simulink model "sampleModel356"  (R2021b)
settings: Solver=VariableStepAuto  StartTime=0.0  StopTime=10.0  RelTol=1e-3
libraries: simulink x5, slpidlib x1
settings Model: Creator=user  LastModifiedBy=user

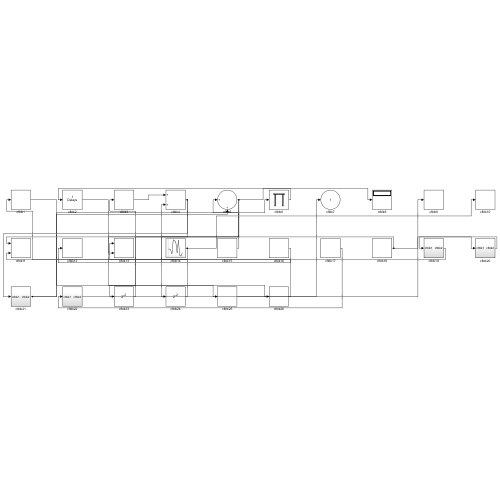
[thumbnail: Simulink's stored preview of the top-level diagram]
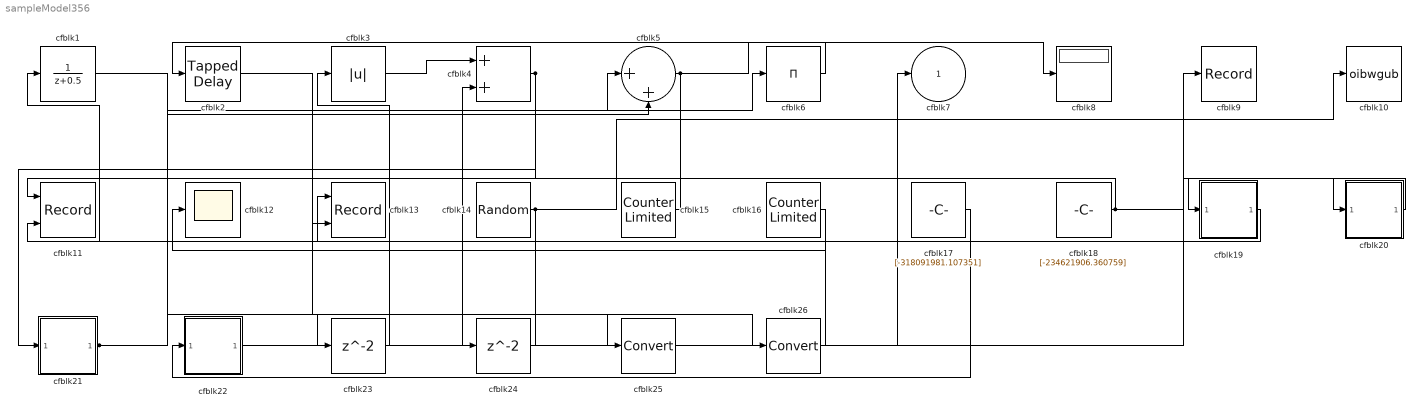
== system sampleModel356 ==
  cfblk1 : DiscreteTransferFcn  SampleTime=1
  cfblk10 : ToWorkspace  VariableName=oibwgub  SaveFormat=Timeseries  SampleTime=-1
  cfblk11 : Record  FileSettingsInternal="{\"entries\":[{\"content\":{\"excelSettings\":{\"content\":{},\"type\":\"Streamout.ExcelSettings\"}},\"type\":\"Streamout.FileSettingStorage\",\"uuid\":\"f7cf1135-fab7-49b0-b509-b4096393f572\"}],\"packageUris\":[\"http://schema.mathworks.com/mf0/streamout_blocks/R2020a\"],\"version\":\"1.0\"}"  Layout=[1 1]  SignalsInternal="{\"entries\":[{\"content\":{\"signals\":[{\"content\":{\"blockPath\":[\"sampleModel356/cfblk11\"],\"channel\":[],\"dimensions\":[1],\"domain\":\"sampleModel356/cfblk11\",\"lineColor\":\"#a2142f\",\"plots\":[1],\"port\":1,\"sid\":[\"\"],\"signalID\":14870,\"signalName\":\"cfblk18\"},\"type\":\"RecordBlkView.Signal\",\"uuid\":\"d168b0b0-4f10-46dc-9af9-509f06b761f4\"},{\"content\":{\"blockPath\":[\"sampleModel356/cfblk11\"],\"channel\":[],\"dimensions\":[1],\"domain\":\"sampleModel356/cfblk11\",\"lineColor\":\"#139fff\",\"plots\":[1],\"port\":2,\"sid\":[\"\"],\"signalID\":14874,\"signalName\":\"cfblk19\"},\"type\":\"RecordBlkView.Signal\",\"uuid\":\"3ec3915b-5336-4778-a6a6-2cfbcdc7d7d8\"}]},\"type\":\"RecordBlkView.InputSignals\",\"uuid\":\"4694ec6d-5d00-4abc-8da0-1736562e4cc9\"}],\"packageUris\":[\"http://schema.mathworks.com/mf0/streamout_blocks/R2020a\"],\"version\":\"1.0\"}"  VisualizationBindings="{\"xyplotplugin\":{\"info\":[{\"series\":[{\"bindingParametersList\":[{\"parameter\":\"X-Axis\",\"signalID\":14870,\"signalName\":\"cfblk18\"},{\"parameter\":\"Y-Axis\",\"signalID\":14874,\"signalName\":\"cfblk19\"}],\"seriesID\":13210}],\"subplotID\":1}]}}"  CompatibilityTag=XY
  cfblk12 : Scope
  cfblk13 : Record  FileSettingsInternal="{\"entries\":[{\"content\":{\"excelSettings\":{\"content\":{},\"type\":\"Streamout.ExcelSettings\"}},\"type\":\"Streamout.FileSettingStorage\",\"uuid\":\"1e1e8cce-afe3-4879-8cf3-0e8c36288c66\"}],\"packageUris\":[\"http://schema.mathworks.com/mf0/streamout_blocks/R2020a\"],\"version\":\"1.0\"}"  Layout=[1 1]  SignalsInternal="{\"entries\":[{\"content\":{\"signals\":[{\"content\":{\"blockPath\":[\"sampleModel356/cfblk13\"],\"channel\":[],\"dimensions\":[1],\"domain\":\"sampleModel356/cfblk13\",\"lineColor\":\"#a2142f\",\"plots\":[1],\"port\":1,\"sid\":[\"\"],\"signalID\":14858,\"signalName\":\"cfblk14\"},\"type\":\"RecordBlkView.Signal\",\"uuid\":\"6a327e09-5034-4fe2-a7e3-7112f60d3f56\"},{\"content\":{\"blockPath\":[\"sampleModel356/cfblk13\"],\"channel\":[],\"dimensions\":[1],\"domain\":\"sampleModel356/cfblk13\",\"lineColor\":\"#139fff\",\"plots\":[1],\"port\":2,\"sid\":[\"\"],\"signalID\":14862,\"signalName\":\"cfblk4\"},\"type\":\"RecordBlkView.Signal\",\"uuid\":\"5deca270-7dad-429e-a242-3b5b02cfe700\"}]},\"type\":\"RecordBlkView.InputSignals\",\"uuid\":\"a51ef856-a68c-416b-b2a1-fe280d763758\"}],\"packageUris\":[\"http://schema.mathworks.com/mf0/streamout_blocks/R2020a\"],\"version\":\"1.0\"}"  VisualizationBindings="{\"xyplotplugin\":{\"info\":[{\"series\":[{\"bindingParametersList\":[{\"parameter\":\"X-Axis\",\"signalID\":14858,\"signalName\":\"cfblk14\"},{\"parameter\":\"Y-Axis\",\"signalID\":14862,\"signalName\":\"cfblk4\"}],\"seriesID\":15766}],\"subplotID\":1}]}}"  CompatibilityTag=XY
  cfblk14 : RandomNumber  Mean=[15872.946615]  Variance=[24959.344930]  Seed=[933413514.000000]  SampleTime=0.1
  cfblk15 : simulink/Sources/Counter Limited  uplimit=[477.000000]  tsamp=-1
  cfblk16 : simulink/Sources/Counter Limited  uplimit=[515.000000]  tsamp=-1
  cfblk17 : Constant  Value=[-318091981.107351]  SampleTime=1
  cfblk18 : Constant  Value=[-234621906.360759]  SampleTime=1
  cfblk19 : Subsystem
  cfblk2 : simulink/Discrete/Tapped Delay  vinit=0.0  samptime=-1  NumDelays=1  DelayOrder=Oldest  includeCurrent=off
  cfblk20 : Subsystem
  cfblk21 : Subsystem
  cfblk22 : Subsystem
  cfblk23 : Delay  SampleTime=1
  cfblk24 : Delay  SampleTime=1
  cfblk25 : DataTypeConversion
  cfblk26 : DataTypeConversion
  cfblk3 : Abs
  cfblk4 : Sum
  cfblk5 : Sum  Inputs=|++
  cfblk6 : Product  Inputs=*
  cfblk8 : Display
  cfblk9 : Record  FileSettingsInternal="{\"entries\":[{\"content\":{\"excelSettings\":{\"content\":{},\"type\":\"Streamout.ExcelSettings\"}},\"type\":\"Streamout.FileSettingStorage\",\"uuid\":\"394831a3-6f16-480d-90e3-9806f58ee700\"}],\"packageUris\":[\"http://schema.mathworks.com/mf0/streamout_blocks/R2020a\"],\"version\":\"1.0\"}"  SignalsInternal="{\"entries\":[{\"content\":{\"signals\":[{\"content\":{\"blockPath\":[\"sampleModel356/cfblk9\"],\"channel\":[],\"dimensions\":[1],\"domain\":\"sampleModel356/cfblk9\",\"lineColor\":\"#edb120\",\"plots\":[1],\"port\":1,\"sid\":[\"\"],\"signalID\":14866,\"signalName\":\"cfblk25\"},\"type\":\"RecordBlkView.Signal\",\"uuid\":\"7e7b1933-ec16-40c2-a7dc-3907081fd54a\"}]},\"type\":\"RecordBlkView.InputSignals\",\"uuid\":\"25d2bbb5-58e4-4035-93b0-d4b8c4893eb6\"}],\"packageUris\":[\"http://schema.mathworks.com/mf0/streamout_blocks/R2020a\"],\"version\":\"1.0\"}"  VisualizationBindings="{\"sparklinesplugin\":{\"info\":[{\"bindingParametersList\":[],\"subplotID\":1}]}}"
  cfblk7 : Outport
  wires:
  cfblk18/1 -> cfblk11/1, cfblk20/1(cfblk1)
  cfblk6/1 -> cfblk2/1
  cfblk3/1 -> cfblk4/1
  cfblk22/1(cfblk2) -> cfblk7/1
  cfblk14/1 -> cfblk13/1, cfblk10/1
  cfblk17/1 -> cfblk22/1(cfblk1)
  cfblk4/1 -> cfblk21/1(cfblk1), cfblk13/2
  cfblk5/1 -> cfblk8/1, cfblk23/1, cfblk24/1
  cfblk20/1(cfblk2) -> cfblk19/1(cfblk1)
  cfblk16/1 -> cfblk12/1
  cfblk21/1(cfblk2) -> cfblk6/1, cfblk5/2
  cfblk15/1 -> cfblk5/1
  cfblk19/1(cfblk2) -> cfblk11/2
  cfblk23/1 -> cfblk3/1
  cfblk24/1 -> cfblk4/2
  cfblk1/1 -> cfblk25/1
  cfblk25/1 -> cfblk9/1
  cfblk2/1 -> cfblk26/1
  cfblk26/1 -> cfblk1/1

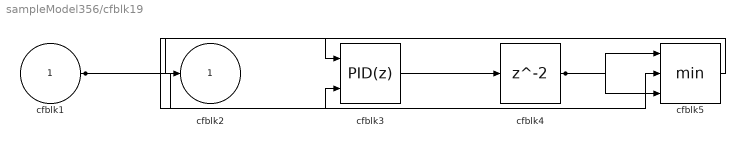
== system sampleModel356/cfblk19 ==
  cfblk1 : Inport
  cfblk3 : slpidlib/PID Controller (2DOF)  Controller=PID  Form=Parallel  TimeDomain=Discrete-time  UseExternalTs=off  SampleTime=1  IntegratorMethod=Forward Euler  FilterMethod=Forward Euler  ControllerParametersSource=internal  P=1  I=1  D=0  UseFilter=on  N=100  b=1  c=1  TunerSelectOption=Transfer Function Based (PID Tuner App)  InitialConditionSource=internal  InitialConditionForIntegrator=0  InitialConditionForFilter=0  DifferentiatorICPrevScaledInput=0  ExternalReset=none  TrackingMode=off  Kt=1  LimitOutput=off  SatLimitsSource=internal  UpperSaturationLimit=inf  LowerSaturationLimit=-inf  LinearizeAsGain=off  AntiWindupMode=none  Kb=1  POutMin=[]  POutMax=[]  IOutMin=[]  IOutMax=[]  DOutMin=[]  DOutMax=[]  NOutMin=[]  NOutMax=[]  bOutMin=[]  bOutMax=[]  cOutMin=[]  cOutMax=[]  SumOutMin=[]  SumOutMax=[]  SaturationOutMin=[]  SaturationOutMax=[]  PParamMin=[]  PParamMax=[]  IParamMin=[]  IParamMax=[]  DParamMin=[]  DParamMax=[]  NParamMin=[]  NParamMax=[]  bParamMin=[]  bParamMax=[]  cParamMin=[]  cParamMax=[]  KbParamMin=[]  KbParamMax=[]  KtParamMin=[]  KtParamMax=[]  KbOutMin=[]  KbOutMax=[]  KtOutMin=[]  KtOutMax=[]  IntegratorOutMin=[]  IntegratorOutMax=[]  FilterOutMin=[]  FilterOutMax=[]  SumI1OutMin=[]  SumI1OutMax=[]  SumI2OutMin=[]  SumI2OutMax=[]  SumI3OutMin=[]  SumI3OutMax=[]  SumI4OutMin=[]  SumI4OutMax=[]  SumDOutMin=[]  SumDOutMax=[]  Sum1OutMin=[]  Sum1OutMax=[]  Sum2OutMin=[]  Sum2OutMax=[]  Sum3OutMin=[]  Sum3OutMax=[]  DifferentiatorOutMin=[]  DifferentiatorOutMax=[]  FilterDiffOutCoefMin=[]  FilterDiffOutCoefMax=[]  ReciprocalOutMin=[]  ReciprocalOutMax=[]  SumDenOutMin=[]  SumDenOutMax=[]  SumNumOutMin=[]  SumNumOutMax=[]  DivideOutMin=[]  DivideOutMax=[]  UdiffTsProdOutMin=[]  UdiffTsProdOutMax=[]  NTsProdOutMin=[]  NTsProdOutMax=[]  UintegralTsProdOutMin=[]  UintegralTsProdOutMax=[]  UngainTsProdOutMin=[]  UngainTsProdOutMax=[]  IntegratorContinuousStateAttributes=''  IntegratorStateMustResolveToSignalObject=off  IntegratorRTWStateStorageClass=Auto  FilterContinuousStateAttributes=''  FilterStateMustResolveToSignalObject=off  FilterRTWStateStorageClass=Auto  ParallelPVariant=InternalParameters  IdealPVariant=Disabled  IVariant=InternalParameters  DVariant=InternalParameters  bVariant=InternalParameters  cVariant=InternalParameters  IntegratorVariant=Discrete  SatVariant=Disabled  AWVariant=Passthrough  PCopyVariant=Disabled  TRVariant=Disabled  FdbkBlocksVariant=Forward  IdealPFdbkVariant=Disabled  SatFdbkVariant=Disabled  DerivativeFilterVariant=ForwardEulerFilter  NVariant=InternalParameters  NCopyVariant=Disabled  FilterICVariant=InternalICsFilter  IntegratorICVariant=InternalICs  ExternalResetVariant=Disabled  TRSumVariant=Passthrough  SumFdbkVariant=Disabled  SumVariant=Sum_PID  TsampFilterVariant=InternalTs  TsampNgainVariant=Passthrough  TsampIntegralVariant=Passthrough  ExternalSaturationOutDataTypeStr=Inherit: Same as second input
      settings: SourceProductBaseCode=SL
  cfblk4 : Delay  SampleTime=1
  cfblk5 : MinMax  Inputs=3
  cfblk2 : Outport
  wires:
  cfblk3/1 -> cfblk4/1
  cfblk4/1 -> cfblk5/1, cfblk5/3
  cfblk1/1 -> cfblk5/2, cfblk3/1, cfblk3/2
  cfblk5/1 -> cfblk2/1

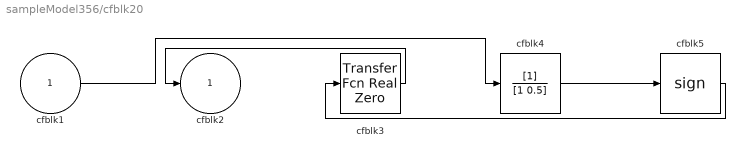
== system sampleModel356/cfblk20 ==
  cfblk1 : Inport
  cfblk3 : simulink/Discrete/Transfer Fcn Real Zero  ZeroZ=0.75  ICPrevInput=0.0  DoSatur=off
      settings: SourceProductBaseCode=SL
  cfblk4 : DiscreteFilter  SampleTime=1
  cfblk5 : Signum
  cfblk2 : Outport
  wires:
  cfblk3/1 -> cfblk2/1
  cfblk4/1 -> cfblk5/1
  cfblk5/1 -> cfblk3/1
  cfblk1/1 -> cfblk4/1

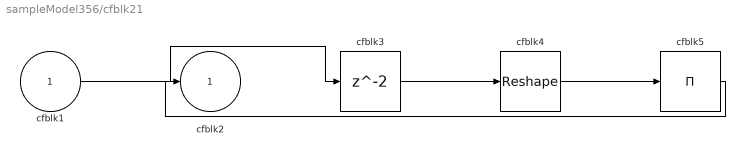
== system sampleModel356/cfblk21 ==
  cfblk1 : Inport
  cfblk3 : Delay  SampleTime=1
  cfblk4 : Reshape
  cfblk5 : Product  Inputs=*
  cfblk2 : Outport
  wires:
  cfblk4/1 -> cfblk5/1
  cfblk3/1 -> cfblk4/1
  cfblk1/1 -> cfblk3/1
  cfblk5/1 -> cfblk2/1

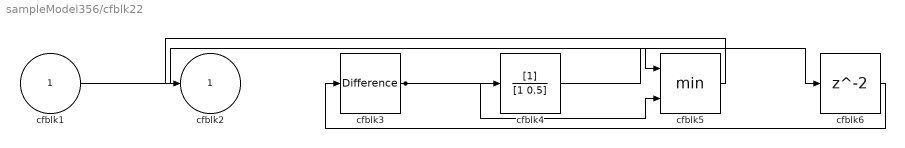
== system sampleModel356/cfblk22 ==
  cfblk1 : Inport
  cfblk3 : simulink/Discrete/Difference  ICPrevInput=0.0  OutMin=[]  OutMax=[]  OutDataTypeStr=Inherit: Inherit via back propagation  OutDataType=fixdt(1, 16)  OutScaling=2^-10  DoSatur=off
  cfblk4 : DiscreteFilter  SampleTime=1
  cfblk5 : MinMax  Inputs=2
  cfblk6 : Delay  SampleTime=1
  cfblk2 : Outport
  wires:
  cfblk1/1 -> cfblk5/1
  cfblk3/1 -> cfblk4/1, cfblk5/2
  cfblk5/1 -> cfblk2/1
  cfblk4/1 -> cfblk6/1
  cfblk6/1 -> cfblk3/1
